simulink library "aerospace"  (R2023b)
settings: Solver=ode45  StartTime=0.0  StopTime=10.0  RelTol=1e-3
undefined symbols (not defined in the file or in its folder): __PRM__SERIALIZED__DATA__, BlockKeywords, convert, Math_Operations_Reshape_convert, Math_Operations_Reshape_reshape, pow
libraries: $bdroot x14
(part 2 of 2)

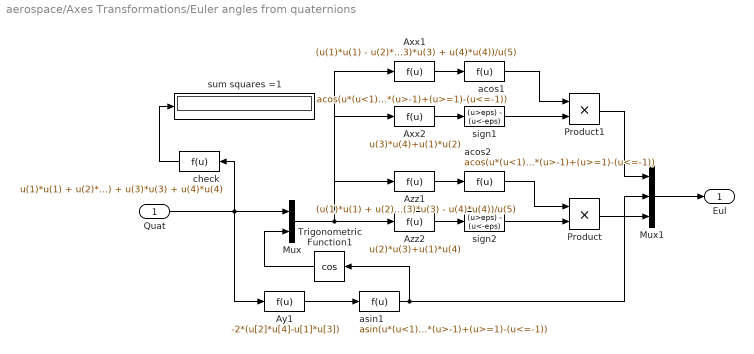
== system aerospace/Axes Transformations/Euler angles from quaternions ==
  Quat : Inport
  Axx1 : Fcn  Expr=(u(1)*u(1) - u(2)*u(2) - u(3)*u(3) + u(4)*u(4))/u(5)
  Axx2 : Fcn  Expr=u(3)*u(4)+u(1)*u(2)
  Ay1 : Fcn  Expr=-2*(u[2]*u[4]-u[1]*u[3])
  Azz1 : Fcn  Expr=(u(1)*u(1) + u(2)*u(2) - u(3)*u(3) - u(4)*u(4))/u(5)
  Azz2 : Fcn  Expr=u(2)*u(3)+u(1)*u(4)
  Mux : Mux  Inputs=2
  Mux1 : Mux  Inputs=3
  Product : Product  InputSameDT=on  RndMeth=Zero  SaturateOnIntegerOverflow=on  OutDataTypeStr=Inherit: Same as first input
  Product1 : Product  InputSameDT=on  RndMeth=Zero  SaturateOnIntegerOverflow=on  OutDataTypeStr=Inherit: Same as first input
  Trigonometric Function1 : Trigonometry  Operator=cos
  acos1 : Fcn  Expr=acos(u*(u<1)*(u>-1)+(u>=1)-(u<=-1))
  acos2 : Fcn  Expr=acos(u*(u<1)*(u>-1)+(u>=1)-(u<=-1))
  "asin1 " : Fcn  Expr=asin(u*(u<1)*(u>-1)+(u>=1)-(u<=-1))
  check : Fcn  Expr=u(1)*u(1) + u(2)*u(2) + u(3)*u(3) + u(4)*u(4)
  sign1 : Fcn  Expr=(u>eps) - (u<-eps)
  sign2 : Fcn  Expr=(u>eps) - (u<-eps)
  sum squares =1 : Display
      settings: Format=long_e
  Eul : Outport  InitialOutput=0  VectorParamsAs1DForOutWhenUnconnected=off
  wires:
  "asin1 "/1 -> Trigonometric Function1/1, Mux1/2
  Mux1/1 -> Eul/1
  Axx1/1 -> acos1/1
  Azz2/1 -> sign2/1
  Azz1/1 -> acos2/1
  Axx2/1 -> sign1/1
  sign2/1 -> Product/2
  acos1/1 -> Product1/1
  check/1 -> sum squares =1/1
  Product1/1 -> Mux1/1
  acos2/1 -> Product/1
  Product/1 -> Mux1/3
  Ay1/1 -> "asin1 "/1
  Trigonometric Function1/1 -> Mux/2
  Mux/1 -> Axx1/1, Azz1/1, Axx2/1, Azz2/1
  Quat/1 -> Ay1/1, check/1, Mux/1
  sign1/1 -> Product1/2

== system aerospace/3DoF Equations of Motion / Equations of Motion (Body Axes)/Gravity ==
  Theta : Inport
  Gain : Gain  Gain=-1  SaturateOnIntegerOverflow=on  OutDataTypeStr=Inherit: Same as input  ParamDataTypeStr=Inherit: Same as input
  Gain2 : Gain  Gain=g  SaturateOnIntegerOverflow=on  OutDataTypeStr=Inherit: Same as input  ParamDataTypeStr=Inherit: Same as input
  Mux : Mux  Inputs=2
  Trigonometric Function : Trigonometry
  Trigonometric Function1 : Trigonometry  Operator=cos
  g : Outport  VectorParamsAs1DForOutWhenUnconnected=off
  wires:
  Theta/1 -> Trigonometric Function1/1, Trigonometric Function/1
  Trigonometric Function/1 -> Gain/1
  Gain/1 -> Mux/1
  Trigonometric Function1/1 -> Mux/2
  Mux/1 -> Gain2/1
  Gain2/1 -> g/1

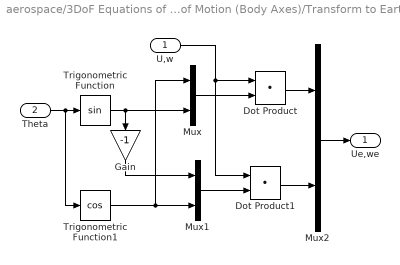
== system aerospace/3DoF Equations of Motion / Equations of Motion (Body Axes)/Transform to Earth Axes ==
  U,w : Inport
  Theta : Inport  Port=2
  Dot Product : DotProduct  OutDataTypeStr=Inherit: Inherit via internal rule
  Dot Product1 : DotProduct  OutDataTypeStr=Inherit: Inherit via internal rule
  Gain : Gain  Gain=-1  SaturateOnIntegerOverflow=on  OutDataTypeStr=Inherit: Same as input  ParamDataTypeStr=Inherit: Same as input
  Mux : Mux  Inputs=2
  Mux1 : Mux  Inputs=2
  Mux2 : Mux  Inputs=2
  Trigonometric Function : Trigonometry
  Trigonometric Function1 : Trigonometry  Operator=cos
  Ue,we : Outport  VectorParamsAs1DForOutWhenUnconnected=off
  wires:
  Trigonometric Function1/1 -> Mux/1, Mux1/2
  Mux1/1 -> Dot Product1/2
  Dot Product/1 -> Mux2/1
  Dot Product1/1 -> Mux2/2
  Mux2/1 -> Ue,we/1
  Mux/1 -> Dot Product/2
  U,w/1 -> Dot Product/1, Dot Product1/1
  Theta/1 -> Trigonometric Function/1, Trigonometric Function1/1
  Trigonometric Function/1 -> Gain/1, Mux/2
  Gain/1 -> Mux1/1

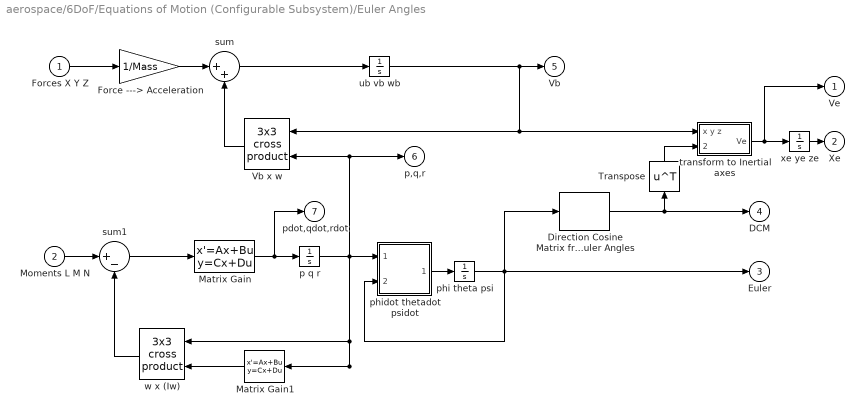
== system aerospace/6DoF/Equations of Motion (Configurable Subsystem)/Euler Angles ==
  Forces X Y Z : Inport
  Moments L M N : Inport  Port=2
  Direction Cosine Matrix from Euler Angles : $bdroot/Axes Transformations/Direction Cosine Matrix from Euler Angles
  Force ---> Acceleration : Gain  Gain=1/Mass  SaturateOnIntegerOverflow=on  OutDataTypeStr=Inherit: Same as input  ParamDataTypeStr=Inherit: Same as input
  Matrix Gain : StateSpace  A=[]  B=[]  C=[]  D=K  InitialCondition=0  mask(Matrix Gain){K=inv(Inertia)}
      mask prompts: K "Gain matrix:"
      mask help: Matrix Gain.
      mask Help: Multiplies input vector by entered matrix to produce output vector (y=Au).
      mask Display: disp('Inertia^(-1)')
  Matrix Gain1 : StateSpace  A=[]  B=[]  C=[]  D=K  InitialCondition=0  mask(Matrix Gain){K=Inertia}
      mask prompts: K "Gain matrix:"
      mask help: Matrix Gain.
      mask Help: Multiplies input vector by entered matrix to produce output vector (y=Au).
      mask Display: disp('Inertia')
  Transpose : Math  Operator=transpose  SignedPower=on
  Vb x w : $bdroot/Axes Transformations/3x3 cross product
  p q r : Integrator  InitialCondition=pm_0
  phi theta psi : Integrator  InitialCondition=eul_0
  phidot thetadot psidot : Subsystem
  sum : Sum  Inputs=|++  InputSameDT=on  SaturateOnIntegerOverflow=on  OutDataTypeStr=Inherit: Same as first input
  sum1 : Sum  Inputs=|+-  InputSameDT=on  SaturateOnIntegerOverflow=on  OutDataTypeStr=Inherit: Same as first input
  "transform to Inertial axes " : Subsystem  mask(Vector Transformation){}
      mask Display: disp('L_EB')
  ub vb wb : Integrator  InitialCondition=Vm_0
  w x (Iw) : $bdroot/Axes Transformations/3x3 cross product
  xe ye ze : Integrator  InitialCondition=xme_0
  Ve : Outport  InitialOutput=0  VectorParamsAs1DForOutWhenUnconnected=off
  Xe : Outport  Port=2  InitialOutput=0  VectorParamsAs1DForOutWhenUnconnected=off
  Euler : Outport  Port=3  InitialOutput=0  VectorParamsAs1DForOutWhenUnconnected=off
  DCM : Outport  Port=4  InitialOutput=0  VectorParamsAs1DForOutWhenUnconnected=off
  Vb : Outport  Port=5  InitialOutput=0  VectorParamsAs1DForOutWhenUnconnected=off
  p,q,r : Outport  Port=6  InitialOutput=0  VectorParamsAs1DForOutWhenUnconnected=off
  pdot,qdot,rdot : Outport  Port=7  InitialOutput=0  VectorParamsAs1DForOutWhenUnconnected=off
  wires:
  Transpose/1 -> "transform to Inertial axes "/2(transform coefficients)
  Direction Cosine Matrix from Euler Angles/1 -> DCM/1, Transpose/1
  Force ---> Acceleration/1 -> sum/1
  Vb x w/1 -> sum/2
  Forces X Y Z/1 -> Force ---> Acceleration/1
  Matrix Gain/1 -> pdot,qdot,rdot/1, p q r/1
  w x (Iw)/1 -> sum1/2
  Matrix Gain1/1 -> w x (Iw)/2
  Moments L M N/1 -> sum1/1
  sum1/1 -> Matrix Gain/1
  p q r/1 -> w x (Iw)/1, phidot thetadot psidot/1(p q r), Matrix Gain1/1, p,q,r/1, Vb x w/2
  "transform to Inertial axes "/1(Ve) -> Ve/1, xe ye ze/1
  xe ye ze/1 -> Xe/1
  sum/1 -> ub vb wb/1
  ub vb wb/1 -> "transform to Inertial axes "/1(x y z), Vb x w/1, Vb/1
  phi theta psi/1 -> Direction Cosine Matrix from Euler Angles/1, phidot thetadot psidot/2(phi theta psi), Euler/1
  phidot thetadot psidot/1(phidot thetadot psi) -> phi theta psi/1

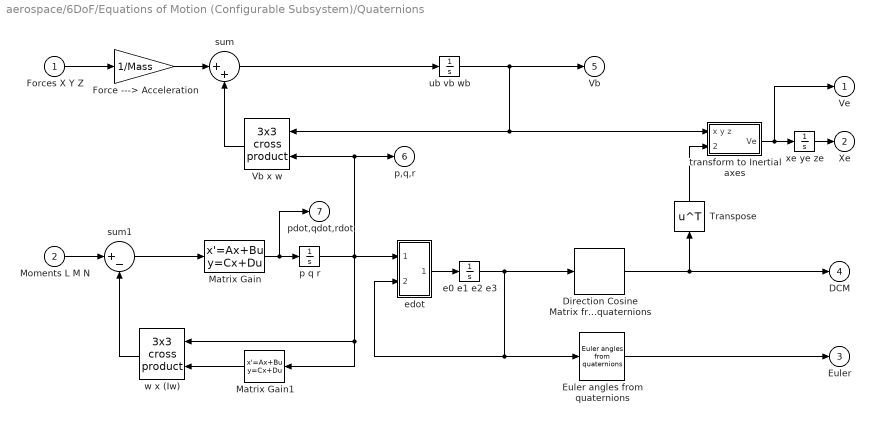
== system aerospace/6DoF/Equations of Motion (Configurable Subsystem)/Quaternions ==
  Forces X Y Z : Inport
  Moments L M N : Inport  Port=2
  Direction Cosine Matrix from quaternions : $bdroot/Axes Transformations/Direction Cosine Matrix from quaternions
  Euler angles from quaternions : $bdroot/Axes Transformations/Euler angles from quaternions
  Force ---> Acceleration : Gain  Gain=1/Mass  SaturateOnIntegerOverflow=on  OutDataTypeStr=Inherit: Same as input  ParamDataTypeStr=Inherit: Same as input
  Matrix Gain : StateSpace  A=[]  B=[]  C=[]  D=K  InitialCondition=0  mask(Matrix Gain){K=inv(Inertia)}
      mask prompts: K "Gain matrix:"
      mask help: Matrix Gain.
      mask Help: Multiplies input vector by entered matrix to produce output vector (y=Au).
      mask Display: disp('Inertia^(-1)')
  Matrix Gain1 : StateSpace  A=[]  B=[]  C=[]  D=K  InitialCondition=0  mask(Matrix Gain){K=Inertia}
      mask prompts: K "Gain matrix:"
      mask help: Matrix Gain.
      mask Help: Multiplies input vector by entered matrix to produce output vector (y=Au).
      mask Display: disp('Inertia')
  Transpose : Math  Operator=transpose  SignedPower=on
  Vb x w : $bdroot/Axes Transformations/3x3 cross product
  e0 e1 e2 e3 : Integrator  InitialCondition=[e0_0 e1_0 e2_0 e3_0]
  edot : Subsystem
  p q r : Integrator  InitialCondition=pm_0
  sum : Sum  Inputs=|++  InputSameDT=on  SaturateOnIntegerOverflow=on  OutDataTypeStr=Inherit: Same as first input
  sum1 : Sum  Inputs=|+-  InputSameDT=on  SaturateOnIntegerOverflow=on  OutDataTypeStr=Inherit: Same as first input
  "transform to Inertial axes " : Subsystem  mask(Vector Transformation){}
      mask Display: disp('L_EB')
  ub vb wb : Integrator  InitialCondition=Vm_0
  w x (Iw) : $bdroot/Axes Transformations/3x3 cross product
  xe ye ze : Integrator  InitialCondition=xme_0
  Ve : Outport  InitialOutput=0  VectorParamsAs1DForOutWhenUnconnected=off
  Xe : Outport  Port=2  InitialOutput=0  VectorParamsAs1DForOutWhenUnconnected=off
  Euler : Outport  Port=3  InitialOutput=0  VectorParamsAs1DForOutWhenUnconnected=off
  DCM : Outport  Port=4  InitialOutput=0  VectorParamsAs1DForOutWhenUnconnected=off
  Vb : Outport  Port=5  InitialOutput=0  VectorParamsAs1DForOutWhenUnconnected=off
  p,q,r : Outport  Port=6  InitialOutput=0  VectorParamsAs1DForOutWhenUnconnected=off
  pdot,qdot,rdot : Outport  Port=7  InitialOutput=0  VectorParamsAs1DForOutWhenUnconnected=off
  wires:
  Transpose/1 -> "transform to Inertial axes "/2(transform coefficients)
  "transform to Inertial axes "/1(Ve) -> Ve/1, xe ye ze/1
  xe ye ze/1 -> Xe/1
  Force ---> Acceleration/1 -> sum/1
  sum/1 -> ub vb wb/1
  Vb x w/1 -> sum/2
  Forces X Y Z/1 -> Force ---> Acceleration/1
  ub vb wb/1 -> "transform to Inertial axes "/1(x y z), Vb x w/1, Vb/1
  Direction Cosine Matrix from quaternions/1 -> DCM/1, Transpose/1
  Matrix Gain/1 -> pdot,qdot,rdot/1, p q r/1
  Euler angles from quaternions/1 -> Euler/1
  e0 e1 e2 e3/1 -> edot/2(in_2), Euler angles from quaternions/1, Direction Cosine Matrix from quaternions/1
  edot/1(out_1) -> e0 e1 e2 e3/1
  w x (Iw)/1 -> sum1/2
  Matrix Gain1/1 -> w x (Iw)/2
  Moments L M N/1 -> sum1/1
  sum1/1 -> Matrix Gain/1
  p q r/1 -> w x (Iw)/1, Matrix Gain1/1, p,q,r/1, Vb x w/2, edot/1(in_1)

== system aerospace/6DoF/Euler Angles/phidot thetadot psidot ==
  p q r : Inport
  phi theta psi : Inport  Port=2
  Mux1 : Mux  Inputs=[3 3]
  Mux2 : Mux  Inputs=3
  phidot : Fcn  Expr=u[1]+u[2]*sin(u[4])*tan(u[5])+u[3]*cos(u[4])*tan(u[5])
  psidot : Fcn  Expr=u[2]*sin(u[4])/cos(u[5])+u[3]*cos(u[4])/cos(u[5])
  thetadot : Fcn  Expr=u[2]*cos(u[4])-u[3]*sin(u[4])
  phidot thetadot psi : Outport  InitialOutput=0  VectorParamsAs1DForOutWhenUnconnected=off
  wires:
  Mux1/1 -> psidot/1, phidot/1, thetadot/1
  p q r/1 -> Mux1/1
  phi theta psi/1 -> Mux1/2
  psidot/1 -> Mux2/3
  thetadot/1 -> Mux2/2
  phidot/1 -> Mux2/1
  Mux2/1 -> phidot thetadot psi/1

== system aerospace/6DoF/Euler Angles/transform to Inertial axes  ==
  x y z : Inport
  transform coefficients : Inport  Port=2
  Product : Product  Multiplication=Matrix(*)  InputSameDT=on  RndMeth=Zero  SaturateOnIntegerOverflow=on  OutDataTypeStr=Inherit: Same as first input
  Ve : Outport  InitialOutput=0  VectorParamsAs1DForOutWhenUnconnected=off
  wires:
  x y z/1 -> Product/2
  transform coefficients/1 -> Product/1
  Product/1 -> Ve/1

== system aerospace/6DoF/Quaternions/edot ==
  in_1 : Inport
  in_2 : Inport  Port=2
  Gain : Gain  Gain=k_quat  SaturateOnIntegerOverflow=on  OutDataTypeStr=Inherit: Same as input  ParamDataTypeStr=Inherit: Same as input
  Mux1 : Mux  Inputs=[3 4 1]
  Mux2 : Mux
  e0dot : Fcn  Expr=-0.5 * ( u[5]*u[1]+u[6]*u[2]+u[7]*u[3] ) + u[8]*u[4]
  e1dot : Fcn  Expr=0.5 * ( u[4]*u[1]+u[6]*u[3]-u[7]*u[2] ) + u[8]*u[5]
  e2dot : Fcn  Expr=0.5 * ( u[4]*u[2]+u[7]*u[1]-u[5]*u[3] ) + u[8]*u[6]
  e3dot : Fcn  Expr=0.5 * ( u[4]*u[3]+u[5]*u[2]-u[6]*u[1] ) + u[8]*u[7]
  lambda : Fcn  Expr=1-( pow(u[1],2) + pow(u[2],2) + pow(u[3],2) + pow(u[4],2) )
  out_1 : Outport  InitialOutput=0  VectorParamsAs1DForOutWhenUnconnected=off
  wires:
  Mux2/1 -> out_1/1
  in_1/1 -> Mux1/1
  e0dot/1 -> Mux2/1
  e1dot/1 -> Mux2/2
  e2dot/1 -> Mux2/3
  Mux1/1 -> e0dot/1, e1dot/1, e2dot/1, e3dot/1
  e3dot/1 -> Mux2/4
  lambda/1 -> Gain/1
  Gain/1 -> Mux1/3
  in_2/1 -> lambda/1, Mux1/2

== system aerospace/6DoF/Quaternions/transform to Inertial axes  ==
  x y z : Inport
  transform coefficients : Inport  Port=2
  Product : Product  Multiplication=Matrix(*)  InputSameDT=on  RndMeth=Zero  SaturateOnIntegerOverflow=on  OutDataTypeStr=Inherit: Same as first input
  Ve : Outport  InitialOutput=0  VectorParamsAs1DForOutWhenUnconnected=off
  wires:
  Product/1 -> Ve/1
  transform coefficients/1 -> Product/1
  x y z/1 -> Product/2

== system aerospace/6DoF/Equations of Motion (Configurable Subsystem)/Euler Angles/phidot thetadot psidot ==
  p q r : Inport
  phi theta psi : Inport  Port=2
  Mux1 : Mux  Inputs=[3 3]
  Mux2 : Mux  Inputs=3
  phidot : Fcn  Expr=u[1]+u[2]*sin(u[4])*tan(u[5])+u[3]*cos(u[4])*tan(u[5])
  psidot : Fcn  Expr=u[2]*sin(u[4])/cos(u[5])+u[3]*cos(u[4])/cos(u[5])
  thetadot : Fcn  Expr=u[2]*cos(u[4])-u[3]*sin(u[4])
  phidot thetadot psi : Outport  InitialOutput=0  VectorParamsAs1DForOutWhenUnconnected=off
  wires:
  Mux2/1 -> phidot thetadot psi/1
  phidot/1 -> Mux2/1
  thetadot/1 -> Mux2/2
  psidot/1 -> Mux2/3
  phi theta psi/1 -> Mux1/2
  p q r/1 -> Mux1/1
  Mux1/1 -> thetadot/1, phidot/1, psidot/1

== system aerospace/6DoF/Equations of Motion (Configurable Subsystem)/Euler Angles/transform to Inertial axes  ==
  x y z : Inport
  transform coefficients : Inport  Port=2
  Product : Product  Multiplication=Matrix(*)  InputSameDT=on  RndMeth=Zero  SaturateOnIntegerOverflow=on  OutDataTypeStr=Inherit: Same as first input
  Ve : Outport  InitialOutput=0  VectorParamsAs1DForOutWhenUnconnected=off
  wires:
  Product/1 -> Ve/1
  transform coefficients/1 -> Product/1
  x y z/1 -> Product/2

== system aerospace/6DoF/Equations of Motion (Configurable Subsystem)/Quaternions/edot ==
  in_1 : Inport
  in_2 : Inport  Port=2
  Gain : Gain  Gain=k_quat  SaturateOnIntegerOverflow=on  OutDataTypeStr=Inherit: Same as input  ParamDataTypeStr=Inherit: Same as input
  Mux1 : Mux  Inputs=[3 4 1]
  Mux2 : Mux
  e0dot : Fcn  Expr=-0.5 * ( u[5]*u[1]+u[6]*u[2]+u[7]*u[3] ) + u[8]*u[4]
  e1dot : Fcn  Expr=0.5 * ( u[4]*u[1]+u[6]*u[3]-u[7]*u[2] ) + u[8]*u[5]
  e2dot : Fcn  Expr=0.5 * ( u[4]*u[2]+u[7]*u[1]-u[5]*u[3] ) + u[8]*u[6]
  e3dot : Fcn  Expr=0.5 * ( u[4]*u[3]+u[5]*u[2]-u[6]*u[1] ) + u[8]*u[7]
  lambda : Fcn  Expr=1-( pow(u[1],2) + pow(u[2],2) + pow(u[3],2) + pow(u[4],2) )
  out_1 : Outport  InitialOutput=0  VectorParamsAs1DForOutWhenUnconnected=off
  wires:
  in_2/1 -> Mux1/2, lambda/1
  Gain/1 -> Mux1/3
  lambda/1 -> Gain/1
  e3dot/1 -> Mux2/4
  Mux1/1 -> e3dot/1, e2dot/1, e1dot/1, e0dot/1
  e2dot/1 -> Mux2/3
  e1dot/1 -> Mux2/2
  e0dot/1 -> Mux2/1
  in_1/1 -> Mux1/1
  Mux2/1 -> out_1/1

== system aerospace/6DoF/Equations of Motion (Configurable Subsystem)/Quaternions/transform to Inertial axes  ==
  x y z : Inport
  transform coefficients : Inport  Port=2
  Product : Product  Multiplication=Matrix(*)  InputSameDT=on  RndMeth=Zero  SaturateOnIntegerOverflow=on  OutDataTypeStr=Inherit: Same as first input
  Ve : Outport  InitialOutput=0  VectorParamsAs1DForOutWhenUnconnected=off
  wires:
  x y z/1 -> Product/2
  transform coefficients/1 -> Product/1
  Product/1 -> Ve/1
